simulink model "Practica7"  (R2020b)
settings: Solver=VariableStepAuto  StartTime=0.0  StopTime=10.0  RelTol=1e-3
undefined symbols (not defined in the file or in its folder): DiscIntNeverNeededParam, sigbuilder_block
libraries: simulink x9
settings Model: Creator=Jordan  LastModifiedBy=Jordan

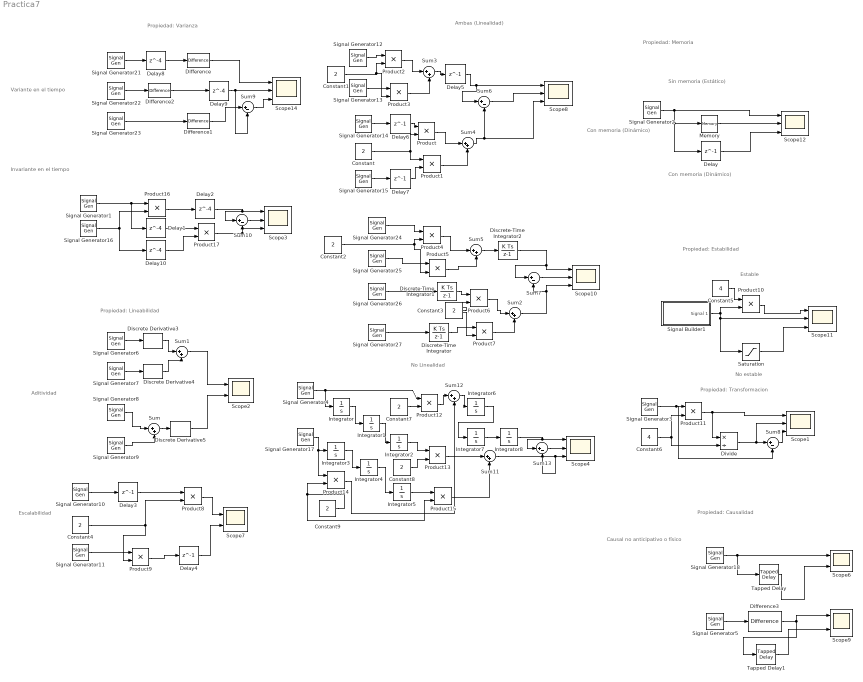
== system Practica7 ==
  note: Invariante en el tiempo
  note: Variante en el tiempo
  note: Propiedad: Varianza
  note: Con memoria (Dinámico)
  note: Sin memoria (Estático)
  note: Con memoria (Dinámico)
  note: Propiedad: Memoria
  note: No estable
  note: Estable
  note: Aditividad
  note: Ambas (Linealidad)
  note: Escalabilidad
  note: Causal no anticipativo o físico
  note: Propiedad: Causalidad
  note: Propiedad: Lineabilidad
  note: Propiedad: Estabilidad
  note: No Linealidad
  note: Propiedad: Transformacion
  Constant{,1..4,7..9} (8 alike) : Constant  Value=2
  Constant5 : Constant  Value=4
  Constant6 : Constant  Value=4
  Delay{,3..7} (6 alike) : Delay  DelayLength=1  InitialCondition=0
  Delay1 : Delay  DelayLength=4
  Delay10 : Delay  DelayLength=4
  Delay2 : Delay  DelayLength=4
  Delay8 : Delay  DelayLength=4  InitialCondition=0
  Delay9 : Delay  DelayLength=4  InitialCondition=0
  Difference{,1..3} (4 alike) : simulink/Discrete/Difference  ICPrevInput=0.0  OutMin=[]  OutMax=[]  OutDataType=fixdt(1, 16)  OutScaling=2^-10  DoSatur=off
  Discrete Derivative3 : simulink/Discrete/Discrete Derivative  gainval=1.0  ICPrevScaledInput=0.0  OutMin=[]  OutMax=[]  OutDataType=fixdt(1, 16)  OutScaling=2^-10  DoSatur=off
  Discrete Derivative4 : simulink/Discrete/Discrete Derivative  gainval=1.0  ICPrevScaledInput=0.0  OutMin=[]  OutMax=[]  OutDataType=fixdt(1, 16)  OutScaling=2^-10  DoSatur=off
  Discrete Derivative5 : simulink/Discrete/Discrete Derivative  gainval=1.0  ICPrevScaledInput=0.0  OutMin=[]  OutMax=[]  OutDataType=fixdt(1, 16)  OutScaling=2^-10  DoSatur=off
  Discrete-Time Integrator : DiscreteIntegrator  SampleTime=-1  ICPrevOutput=DiscIntNeverNeededParam  ICPrevScaledInput=DiscIntNeverNeededParam
  Discrete-Time Integrator1 : DiscreteIntegrator  SampleTime=-1  ICPrevOutput=DiscIntNeverNeededParam  ICPrevScaledInput=DiscIntNeverNeededParam
  Discrete-Time Integrator2 : DiscreteIntegrator  SampleTime=-1  ICPrevOutput=DiscIntNeverNeededParam  ICPrevScaledInput=DiscIntNeverNeededParam
  Divide : Product  Inputs=*/
  Integrator : Integrator
  Integrator1 : Integrator  InitialCondition=1
  Integrator2 : Integrator  InitialCondition=1.05
  Integrator3 : Integrator
  Integrator4 : Integrator  InitialCondition=1
  Integrator5 : Integrator  InitialCondition=1.05
  Integrator6 : Integrator
  Integrator7 : Integrator  InitialCondition=1
  Integrator8 : Integrator  InitialCondition=1.05
  Memory : Memory
  Product{,1..17} (18 alike) : Product
  Saturation : Saturate
  Scope{1,3..4,8,10..12,14} (8 alike) : Scope  NumInputPorts=3
  Scope{2,6..7,9} (4 alike) : Scope  NumInputPorts=2
  Signal Generator{1..2,4,17,24..27} (8 alike) : SignalGenerator  WaveForm=square  Units=rad/sec
  Signal Generator{3,5..16,18,21..23} (17 alike) : SignalGenerator  Units=rad/sec
  Signal Builder1 : Subsystem  Tag=STV Subsys  LoadFcn=sigbuilder_block('load');  StartFcn=sigbuilder_block('start');  StopFcn=sigbuilder_block('stop');  ClipboardFcn=sigbuilder_block('clipboard');  mask(Sigbuilder block){tuvar=[0:10]}
      mask help: Simulink:masks:SigbuilderBlock_MD
      mask init:
      | if ~strcmp(get_param(bdroot(gcbh),'SimulationStatus'),'stopped') tuvar = sigbuilder_block('maskInit'); end
      settings: CopyFcn=sigbuilder_block('copy');  DeleteFcn=sigbuilder_block('delete');  ModelCloseFcn=sigbuilder_block('modelClose');  PreSaveFcn=sigbuilder_block('preSave');  PauseFcn=sigbuilder_block('pause');  ContinueFcn=sigbuilder_block('continue');  NameChangeFcn=sigbuilder_block('namechange');  OpenFcn=sigbuilder_block('open',[427.5 90 550.5 400.5 ]);  CloseFcn=sigbuilder_block('close');
      mask Display: plot(0, 0, 100, 100,[2, 2, 32, 32, 2], [68, 8, 8, 68, 68],[32, 2], [38, 38], [32, 19, 2],[53, 60, 44], [32, 17, 17, 2],[16, 16, 31, 31]);txt = getActiveGroup(gcbh);text(2, 100, txt,'verticalAlignment', 'top');
  Sum{,1..5,11..12} (8 alike) : Sum  Inputs=|++
  Sum{6..10,13} (6 alike) : Sum  Inputs=|+-
  Tapped Delay : simulink/Discrete/Tapped Delay  vinit=0.0  samptime=-1  NumDelays=5  DelayOrder=Oldest  includeCurrent=off
  Tapped Delay1 : simulink/Discrete/Tapped Delay  vinit=0.0  samptime=-1  NumDelays=5  DelayOrder=Oldest  includeCurrent=off
  wires:
  Delay8/1 -> Difference/1
  Difference/1 -> Scope14/1
  Signal Generator21/1 -> Delay8/1
  Delay9/1 -> Scope14/2, Sum9/2
  Difference2/1 -> Delay9/1
  Signal Generator23/1 -> Difference1/1
  Signal Generator22/1 -> Difference2/1
  Product10/1 -> Scope11/1
  Signal Builder1/1(Signal 1) -> Scope11/2, Saturation/1, Product10/2
  Sum2/1 -> Scope10/3, Sum7/2
  Sum5/1 -> Discrete-Time Integrator2/1
  Product9/1 -> Delay4/1
  Discrete Derivative5/1 -> Scope2/2
  Signal Generator6/1 -> Discrete Derivative3/1
  Discrete Derivative3/1 -> Sum1/1
  Signal Generator8/1 -> Sum/1
  Signal Generator14/1 -> Delay6/1
  Discrete Derivative4/1 -> Sum1/2
  Sum1/1 -> Scope2/1
  Signal Generator26/1 -> Discrete-Time Integrator1/1
  Product8/1 -> Scope7/1
  Sum/1 -> Discrete Derivative5/1
  Signal Generator27/1 -> Discrete-Time Integrator/1
  Signal Generator15/1 -> Delay7/1
  Sum3/1 -> Delay5/1
  Product/1 -> Sum4/1
  Product5/1 -> Sum5/2
  Signal Generator9/1 -> Sum/2
  Sum4/1 -> Sum6/2, Scope8/3
  Product1/1 -> Sum4/2
  Delay6/1 -> Product/1
  Delay4/1 -> Scope7/2
  Signal Generator10/1 -> Delay3/1
  Signal Generator7/1 -> Discrete Derivative4/1
  Discrete-Time Integrator2/1 -> Scope10/1, Sum7/1
  Delay7/1 -> Product1/2
  Delay5/1 -> Sum6/1, Scope8/1
  Sum6/1 -> Scope8/2
  Constant/1 -> Product/2, Product1/1
  Signal Generator13/1 -> Product3/1
  Product2/1 -> Sum3/1
  Product3/1 -> Sum3/2
  Constant1/1 -> Product2/2, Product3/2
  Signal Generator12/1 -> Product2/1
  Signal Generator24/1 -> Product4/1
  Product4/1 -> Sum5/1
  Constant2/1 -> Product5/2, Product4/2
  Signal Generator25/1 -> Product5/1
  Product7/1 -> Sum2/2
  Product6/1 -> Sum2/1
  Constant3/1 -> Product7/2, Product6/2
  Discrete-Time Integrator/1 -> Product7/1
  Discrete-Time Integrator1/1 -> Product6/1
  Constant4/1 -> Product8/2, Product9/2
  Signal Generator11/1 -> Product9/1
  Delay3/1 -> Product8/1
  Tapped Delay1/1 -> Scope9/2
  Signal Generator18/1 -> Tapped Delay/1, Scope6/1
  Difference3/1 -> Tapped Delay1/1, Scope9/1
  Tapped Delay/1 -> Scope6/2
  Signal Generator5/1 -> Difference3/1
  Constant5/1 -> Product10/1
  Sum7/1 -> Scope10/2
  Saturation/1 -> Scope11/3
  Signal Generator2/1 -> Scope12/1, Memory/1, Delay/1
  Memory/1 -> Scope12/2
  Delay/1 -> Scope12/3
  Signal Generator3/1 -> Sum8/2, Product11/1
  Constant6/1 -> Divide/2, Product11/2
  Product11/1 -> Divide/1, Scope1/1
  Divide/1 -> Sum8/1, Scope1/2
  Sum8/1 -> Scope1/3
  Difference1/1 -> Sum9/1
  Sum9/1 -> Scope14/3
  Signal Generator16/1 -> Delay10/1, Product16/2
  Product17/1 -> Scope3/3, Sum10/2
  Signal Generator1/1 -> Delay1/1, Product16/1
  Delay1/1 -> Product17/1
  Delay2/1 -> Sum10/1, Scope3/1
  Delay10/1 -> Product17/2
  Product16/1 -> Delay2/1
  Sum10/1 -> Scope3/2
  Integrator5/1 -> Product15/1
  Signal Generator17/1 -> Product14/1, Integrator3/1
  Integrator8/1 -> Sum13/1, Scope4/1
  Sum11/1 -> Sum13/2, Scope4/3
  Product14/1 -> Sum12/2
  Sum13/1 -> Scope4/2
  Product12/1 -> Sum12/1
  Product13/1 -> Sum11/1
  Integrator1/1 -> Integrator2/1
  Integrator3/1 -> Integrator4/1
  Integrator4/1 -> Integrator5/1
  Integrator/1 -> Integrator1/1
  Product15/1 -> Sum11/2
  Signal Generator4/1 -> Integrator/1, Product12/1
  Constant7/1 -> Product12/2
  Integrator2/1 -> Product13/1
  Constant8/1 -> Product13/2
  Constant9/1 -> Product14/2, Product15/2
  Sum12/1 -> Integrator6/1
  Integrator6/1 -> Integrator7/1
  Integrator7/1 -> Integrator8/1

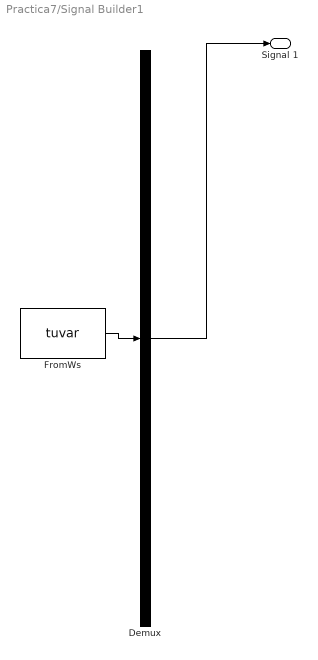
== system Practica7/Signal Builder1 ==
  Demux : Demux  Tag=STV Demux  Outputs=1
      settings: DisplayOption=none
  FromWs : FromWorkspace  Tag=STV FromWs  VariableName=tuvar
      SigBuilderData=|
      | common.afterFinalStr = 'Extrapolate'
      | common.sampleTime = 0
      | dataSet.timeRange = [2 6]
      | dataSet.name = 'Group 1'
      | sbobj.Groups.Name = 'Group 1'
      | sbobj.Groups.Signals.Name = 'Signal 1'
      | sbobj.Groups.Signals.XData = [2 3 3 4 4 5 5 6]
      | sbobj.Groups.Signals.YData = [0 2 0 2 0 2 0 2]
      | sbobj.Groups.TimeRange = [2 6]
  Signal 1 : Outport  Tag=STV Outport
  wires:
  FromWs/1 -> Demux/1
  Demux/1 -> Signal 1/1
